simulink model "GridConnectedPV"  (R2023b)
settings: Solver=ode23t  StartTime=0.0  StopTime=simulation.timeSim  MaxStep=1/(5*solarPlant.switchFrequency)  RelTol=1e-3  AbsTol=1e-3
PreLoadFcn:
  | run('GridConnectedPVData');
undefined symbols (not defined in the file or in its folder): closedLoop, controller, grid, protection, sensor, solarPanel, solarPlant
libraries: nesl_utility x29, simulink x19, fl_lib x18, ee_lib x12, eeTransforms x2, simulink_extras x2, eeRmsMeasurement x1, eeSinusoidalMeasurement x1, slpidlib x1, eePwmGeneratorThreeLevel x1, eePwmGenerator x1
(part 1 of 2)
CloseFcn:
  | try,close(figHandleGridconnectedSolarThreePhase),end
  | clear figHandleGridconnectedSolarThreePhase
  | clear warnState
  | clear simlog_GridConnectedPV
  | 
  | clear solarPanel grid solarPlant sensor controller protection simulation
  | clear inductorDesign closedLoop
  | clear remainingPowerPerString
  | clear simulation  MPPT  powerCircuit
  | clear incrementalConductance perturbationAndObservation
  | clear discrete average continuous
  | clear modelName X U idx t x y X U A B C D G closedLoop
  | clear npts f G magline_h phsline_h presentMPPTVariant presentInverterVariant
  | clear i inverter twoLevel threeLevel geometricMean
  | clear currentLoopPole figAxes
  | clear xout yout tout
  | clear figHandleGridconnectedSolarthreePhase
Description:
  | Three-Phase Grid-Connected Solar Photovoltaic System
  | 
  | %
settings Model: Creator=The MathWorks, Inc.  LastModifiedBy=dy350
settings SolverCC: AlgebraicLoopSolver=TrustRegion
settings DataIOCC: SaveState=on  SignalLogging=off  DSMLogging=off  ReturnWorkspaceOutputs=off
settings OptimizationCC: ReuseModelBlockBuffer=off
settings DebuggingCC: UnconnectedInputMsg=warning  UnconnectedOutputMsg=warning  UnconnectedLineMsg=warning
settings ModelReferenceCC: EnableRefExpFcnMdlSchedulingChecks=on
settings RTWCC: DLArmComputeVersion=19.05
settings SimscapeCC: SimscapeLogType=all  SimscapeLogName=simlog_GridConnectedPV  SimscapeLogLimitData=off

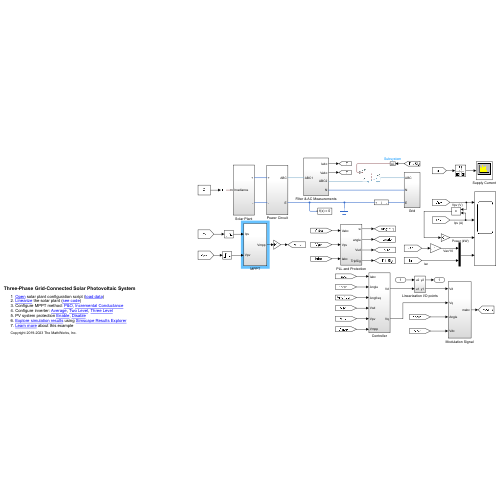
[thumbnail: Simulink's stored preview of the top-level diagram]
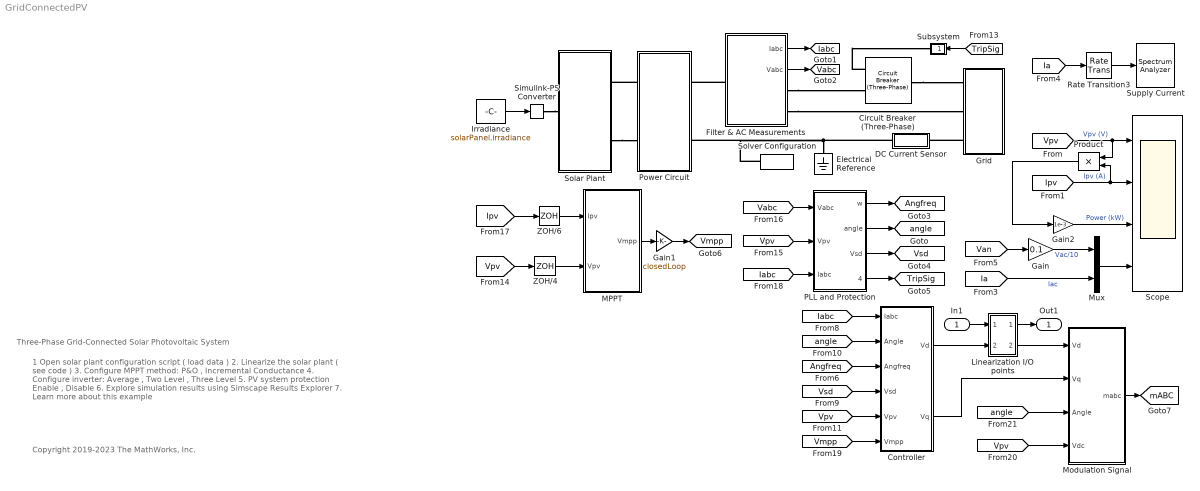
== system GridConnectedPV ==
  note: 1 Open solar plant configuration script ( load data )
      | 2. Linearize the solar plant ( see code )
      | 3. Configure MPPT method: P&O , Incremental Conductance
      | 4. Configure inverter: Average , Two Level , Three Level
      | 5. PV system protection Enable , Disable
      | 6. Explore simulation results using Simscape Results Explorer
      | 7. Learn more about this example
  note: Three-Phase Grid-Connected Solar Photovoltaic System
  note: Copyright 2019-2023 The MathWorks, Inc.
  In1 : Inport
  Circuit Breaker (Three-Phase) : ee_lib/Switches & Breakers/Circuit Breaker (Three-Phase)  R_closed=0.0001 Ohm  G_open=1e-6 1/Ohm  threshold=0.5 V  breaker_behavior=ee.enum.switches.breakerBehavior.zeroCrossingEnable
      settings: InternalSimscapePortConfiguration="{\"Bottom\":[],\"Left\":[{\"id\":\"vT\",\"label\":\"vT\",\"type\":\"input\"},{\"id\":\"N1\",\"label\":\"~1\",\"type\":\"foundation.electrical.three_phase\"}],\"Right\":[{\"id\":\"N2\",\"label\":\"~2\",\"type\":\"foundation.electrical.three_phase\"}],\"Top\":[]}"
  Controller : Subsystem
  DC Current Sensor : Subsystem
      mask Display: disp('i')
  Electrical Reference : fl_lib/Electrical/Electrical Elements/Electrical Reference
  Filter & AC Measurements : Subsystem
  Gain : Gain  Gain=0.1
  Gain1 : Gain  Gain=closedLoop
  Gain2 : Gain  Gain=1e-3
  Grid : Subsystem
  Irradiance : Constant  Value=solarPanel.irradiance
  Linearization I/O points : Subsystem
  MPPT : Subsystem
  Modulation Signal : Subsystem
  Mux : Mux  Inputs=2
  PLL and Protection : Subsystem
  Power Circuit : Subsystem
  Product : Product
  Rate Transition3 : RateTransition  OutPortSampleTime=1/(5*solarPlant.switchFrequency)
  Scope : Scope  NumInputPorts=4
  Simulink-PS Converter : nesl_utility/Simulink-PS Converter  PhysicalDomain=network_engine_domain  SubClassName=ps_input  LeftPortType=input  RightPortType=output  PseudoPeriodic=off  Frequencies=[]  NoiseDistribution=none  NoiseParameters=[]  Unit=1  AffineConversion=off  FilteringAndDerivatives=provide  SimscapeFilterOrder=1  InputFilterTimeConstant=0.001  UdotUserProvided=0
  Solar Plant : Subsystem
  Solver Configuration : nesl_utility/Solver Configuration  PhysicalDomain=network_engine_domain  SubClassName=solver  LeftPortType=input  RightPortType=generic  Tones=[]  Harmonics=[]  SimulateNoise=off  Profile=off  UseLocalSampling=off  EnableSwitchedLinearOptims=on  FrequencyDomain=off  UseCCode=off  RelTol=0.001  AbsTol=1e-06  MinStep=1e-09  ToWorkspace=off  RevertToSquareIcSolve=off  NumHomotopyIterations=100  PhasorMode=off  PhasorModeNumHarmonics=1  ConsistencySolver=NEWTON_FTOL  IndexReductionMethod=DerivativeReplacement  DoDC=off  ResidualTolerance=1e-9  ConsistencyTolSource=GLOBAL  ConsistencyAbsTol=0.001  ConsistencyRelTol=0.001  ConsistencyTolFactor=0.001  UseLocalSolver=off  LocalSolverChoice=NE_TRAPEZOIDAL_ADVANCER  ResolveIndetEquations=on  FunctionEvalNumThread=1  LocalSolverSampleTime=1e-7  DoFixedCost=off  MaxNonlinIter=10  MaxModeIter=2  ComputeImpulses=off  ImpulseIterations=2  LinearAlgebra=auto  LinearAlgebraNumThread=0  EquationFormulation=NE_TIME_EF  DelaysMemoryBudget=1024  AutomaticFiltering=on  FilteringTimeConstant=0.001  PartitionStorageMethod=AS_NEEDED  PartitionMemoryBudget=1024  PartitionMethod=FAST  MultibodyUseLocalSolver=off  MultibodyLocalSolverChoice=ODE1  MultibodyLocalSolverSampleTime=0.001
  Subsystem : Subsystem
  Supply Current : SpectrumAnalyzer  WindowPosition=[1.000000,49.000000,1707.000000,996.000000,]  ScopeFrameLocation=window  SpectrumType=RMS  Method=Welch  SampleRate=100000  PlotAsTwoSidedSpectrum=off  FrequencyScale=Log  AxesScaling=Manual  Span=50000  CenterFrequency=25000  StartFrequency=0  StopFrequency=50000  RBWSource=Property  RBW=9  OverlapPercent=90  AveragingMethod=Running  SpectrumUnits=Vrms  YLimits=[-5.01533311,45.13799799]  ColorLimits=[0.0061790664803535039207,16.888204283875005274]  ShowLegend=on
      settings: OpenAtSimulationStart=off
  ZOH/4 : ZeroOrderHold  SampleTime=solarPlant.timeMPPT
  ZOH/6 : ZeroOrderHold  SampleTime=solarPlant.timeMPPT
  Out1 : Outport  VectorParamsAs1DForOutWhenUnconnected=off
  tag scope: Angfreq=global, Iabc=global, TripSig=global, Vabc=global, Vmpp=global, Vsd=global, angle=global, mABC=global
  wires:
  [Iabc] -> Controller/1(Iabc)
  [Vpv] -> Controller/5(Vpv)
  [Vpv] -> PLL and Protection/2(Vpv)
  In1/1 -> Linearization I/O points/1(u2)
  [Vpv] -> ZOH/4/1
  [angle] -> Modulation Signal/3(Angle)
  Linearization I/O points/1(y2) -> Out1/1
  [TripSig] -> Subsystem/1(i)
  Controller/1(Vd) -> Linearization I/O points/2(u1)
  Controller/2(Vq) -> Modulation Signal/2(Vq)
  Gain/1 -> Mux/1  "Vac/10"
  [Ipv] -> Product/2, Scope/2  "Ipv (A)"
  Filter & AC Measurements/1(Iabc) -> [Iabc]
  MPPT/1(Vmpp) -> Gain1/1
  Modulation Signal/1(mabc) -> [mABC]
  PLL and Protection/3(Vsd) -> [Vsd]
  [Vmpp] -> Controller/6(Vmpp)
  PLL and Protection/2(angle) -> [angle]
  PLL and Protection/4(TripSig) -> [TripSig]
  [Vsd] -> Controller/4(Vsd)
  Rate Transition3/1 -> Supply Current/1
  Filter & AC Measurements/2(Vabc) -> [Vabc]
  PLL and Protection/1(w) -> [Angfreq]
  [Iabc] -> PLL and Protection/3(Iabc)
  [Ia] -> Rate Transition3/1
  [Ipv] -> ZOH/6/1
  [Vpv] -> Modulation Signal/4(Vdc)
  [angle] -> Controller/2(Angle)
  [Angfreq] -> Controller/3(Angfreq)
  [Vabc] -> PLL and Protection/1(Vabc)
  [Van] -> Gain/1
  Mux/1 -> Scope/4
  Linearization I/O points/2(y1) -> Modulation Signal/1(Vd)
  Gain2/1 -> Scope/3  "Power (kW)"
  ZOH/6/1 -> MPPT/1(Ipv)
  [Ia] -> Mux/2  "Iac"
  [Vpv] -> Product/1, Scope/1  "Vpv (V)"
  Product/1 -> Gain2/1
  ZOH/4/1 -> MPPT/2(Vpv)
  Gain1/1 -> [Vmpp]
  Irradiance/1 -> Simulink-PS Converter/1
  connections:
  Electrical Reference/LConn1 -- DC Current Sensor/RConn1 -- Solver Configuration/RConn1 -- Power Circuit/RConn2
  Filter & AC Measurements/RConn1 -- Circuit Breaker (Three-Phase)/LConn2
  Filter & AC Measurements/RConn2 -- Grid/LConn2
  Filter & AC Measurements/LConn1 -- Power Circuit/RConn1
  Power Circuit/LConn1 -- Solar Plant/RConn1
  Grid/LConn3 -- DC Current Sensor/LConn1
  Solar Plant/RConn2 -- Power Circuit/LConn2
  Simulink-PS Converter/RConn1 -- Solar Plant/LConn1
  Circuit Breaker (Three-Phase)/RConn1 -- Grid/LConn1
  Circuit Breaker (Three-Phase)/LConn1 -- Subsystem/RConn1

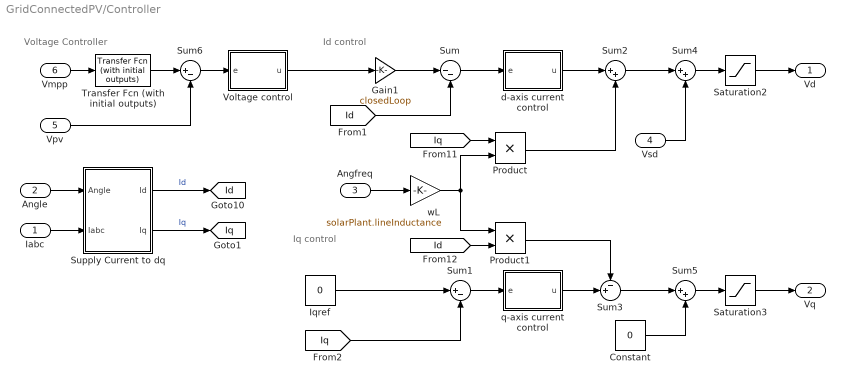
== system GridConnectedPV/Controller ==
  note: Id control
  note: Voltage Controller
  note: Iq control
  Iabc : Inport
  Angle : Inport  Port=2
  Angfreq : Inport  Port=3
  Vsd : Inport  Port=4
  Vpv : Inport  Port=5
  Vmpp : Inport  Port=6
  Constant : Constant  Value=0
  Gain1 : Gain  Gain=closedLoop
  Iqref : Constant  Value=0
  Product : Product
  Product1 : Product
  Saturation2 : Saturate  UpperLimit=controller.currentVoltMax*1.5  LowerLimit=-1*controller.currentVoltMax*1.5
  Saturation3 : Saturate  UpperLimit=controller.currentVoltMax*1.5  LowerLimit=-1*controller.currentVoltMax*1.5
  Sum : Sum  Inputs=|--
  Sum1 : Sum  Inputs=|+-
  Sum2 : Sum  Inputs=|++
  Sum3 : Sum  Inputs=-+|
  Sum4 : Sum  Inputs=|++
  Sum5 : Sum  Inputs=|++
  Sum6 : Sum  Inputs=|+-
  Supply Current to dq : Subsystem
  Transfer Fcn (with initial outputs) : simulink_extras/Additional Linear/Transfer Fcn (with initial outputs)  N=[1]  D="[solarPlant.timeMPPT*50  1]"  Y0=solarPlant.DCMPPTValue  U0=solarPlant.DCMPPTValue
  Voltage control : Subsystem
  d-axis current control : Subsystem
  q-axis current control : Subsystem
  wL : Gain  Gain=solarPlant.lineInductance
  Vd : Outport  VectorParamsAs1DForOutWhenUnconnected=off
  Vq : Outport  Port=2  VectorParamsAs1DForOutWhenUnconnected=off
  tag scope: Id=global, Iq=global
  wires:
  Sum1/1 -> q-axis current control/1(e)
  wL/1 -> Product/2, Product1/1
  [Id] -> Product1/2
  [Iq] -> Product/1
  Product1/1 -> Sum3/1
  Product/1 -> Sum2/2
  Sum3/1 -> Sum5/1
  Sum2/1 -> Sum4/1
  Sum4/1 -> Saturation2/1
  Sum5/1 -> Saturation3/1
  Angfreq/1 -> wL/1
  Constant/1 -> Sum5/2
  Angle/1 -> Supply Current to dq/1(Angle)
  Vpv/1 -> Sum6/2
  Sum/1 -> d-axis current control/1(e)
  [Id] -> Sum/2
  d-axis current control/1(u) -> Sum2/1
  q-axis current control/1(u) -> Sum3/2
  Supply Current to dq/1(Id) -> [Id]  "Id"
  Supply Current to dq/2(Iq) -> [Iq]  "Iq"
  Iabc/1 -> Supply Current to dq/2(Iabc)
  Vsd/1 -> Sum4/2
  Sum6/1 -> Voltage control/1(e)
  Vmpp/1 -> Transfer Fcn (with initial outputs)/1
  Transfer Fcn (with initial outputs)/1 -> Sum6/1
  Saturation3/1 -> Vq/1
  Saturation2/1 -> Vd/1
  Iqref/1 -> Sum1/1
  [Iq] -> Sum1/2
  Voltage control/1(u) -> Gain1/1
  Gain1/1 -> Sum/1

== system GridConnectedPV/DC Current Sensor ==
  note: In the transformerless grid connected PV system, leakage current depends on, PWM technique, DC bus voltage ripple, earth resistance and semi conductor switch switching time. So for accurately estimating the leakage current requires better PWM technique (bipolar PWM), DC bus voltage ripple, semi conductor model and earth resistance.
  Current Sensor : fl_lib/Electrical/Electrical Sensors/Current Sensor
      settings: LogSimulationData=on
  PS-Simulink Converter : nesl_utility/PS-Simulink Converter  PhysicalDomain=network_engine_domain  SubClassName=ps_output  LeftPortType=input  RightPortType=output  PseudoPeriodic=off  Frequencies=[]  VectorFormat=1-D array  Unit=1  AffineConversion=off
  Scope : Scope
  Sensor dynamics : TransferFcn  Numerator=1  Denominator=[1/sensor.samplingFreq 1]
  - : PMIOPort  Side=Left
  + : PMIOPort  Port=2  Side=Right
  wires:
  PS-Simulink Converter/1 -> Sensor dynamics/1
  Sensor dynamics/1 -> Scope/1
  connections:
  Current Sensor/RConn2 -- -/RConn1
  +/RConn1 -- Current Sensor/LConn1
  Current Sensor/RConn1 -- PS-Simulink Converter/LConn1

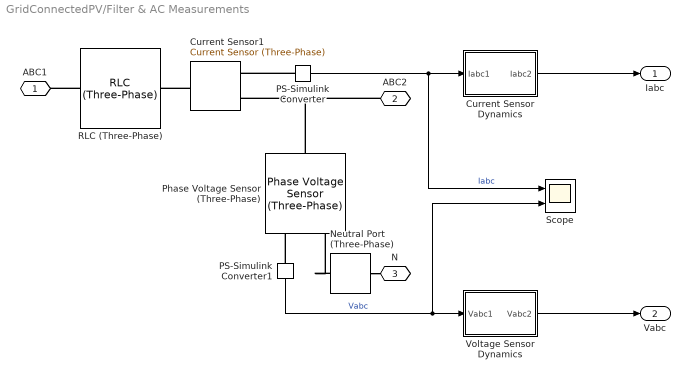
== system GridConnectedPV/Filter & AC Measurements ==
  Current Sensor Dynamics : Subsystem
  Current Sensor1 : ee_lib/Sensors & Transducers/Current Sensor (Three-Phase)
  Neutral Port (Three-Phase) : ee_lib/Connectors & References/Neutral Port (Three-Phase)  G_parasitic=1e-12 1/Ohm
      settings: InternalSimscapePortConfiguration="{\"Bottom\":[],\"Left\":[{\"id\":\"N\",\"label\":\"~\",\"type\":\"foundation.electrical.three_phase\"}],\"Right\":[{\"id\":\"n\",\"label\":\"n\",\"type\":\"foundation.electrical.electrical\"}],\"Top\":[]}"
  PS-Simulink Converter : nesl_utility/PS-Simulink Converter  PhysicalDomain=network_engine_domain  SubClassName=ps_output  LeftPortType=input  RightPortType=output  PseudoPeriodic=off  Frequencies=[]  VectorFormat=1-D array  Unit=inherit  AffineConversion=off
  PS-Simulink Converter1 : nesl_utility/PS-Simulink Converter  PhysicalDomain=network_engine_domain  SubClassName=ps_output  LeftPortType=input  RightPortType=output  PseudoPeriodic=off  Frequencies=[]  VectorFormat=1-D array  Unit=inherit  AffineConversion=off
  Phase Voltage Sensor (Three-Phase) : ee_lib/Sensors & Transducers/Phase Voltage Sensor (Three-Phase)
  RLC (Three-Phase) : ee_lib/Passive/RLC Assemblies/RLC (Three-Phase)  component_structure=4  R=solarPlant.inductorResistance Ohm  L=solarPlant.lineInductance H  C=1e-6 F  R_parasitic=1e-6 Ohm  G_parasitic=1e-6 1/Ohm  IL_specify=on  IL_priority=High  IL=[0, 0, 0] A  IL_nominal_specify=off  IL_nominal_unit=A  IL_nominal_value=1  VC_specify=on  VC_priority=High  VC=[0, 0, 0] V  VC_nominal_specify=off  VC_nominal_unit=V  VC_nominal_value=1
      settings: InternalSimscapePortConfiguration="{\"Bottom\":[],\"Left\":[{\"id\":\"N1\",\"label\":\"~1\",\"type\":\"foundation.electrical.three_phase\"}],\"Right\":[{\"id\":\"N2\",\"label\":\"~2\",\"type\":\"foundation.electrical.three_phase\"}],\"Top\":[]}"
  Scope : Scope  NumInputPorts=2
  Voltage Sensor Dynamics : Subsystem
  ABC1 : PMIOPort  Side=Left
  ABC2 : PMIOPort  Port=2  Side=Right
  N : PMIOPort  Port=3  Side=Right
  Iabc : Outport
  Vabc : Outport  Port=2
  wires:
  PS-Simulink Converter/1 -> Scope/1, Current Sensor Dynamics/1(Iabc1)  "Iabc"
  Current Sensor Dynamics/1(Iabc2) -> Iabc/1
  Voltage Sensor Dynamics/1(Vabc2) -> Vabc/1
  PS-Simulink Converter1/1 -> Scope/2, Voltage Sensor Dynamics/1(Vabc1)  "Vabc"
  connections:
  Current Sensor1/LConn1 -- RLC (Three-Phase)/RConn1
  Phase Voltage Sensor (Three-Phase)/LConn1 -- ABC2/RConn1 -- Current Sensor1/RConn2
  PS-Simulink Converter/LConn1 -- Current Sensor1/RConn1
  PS-Simulink Converter1/LConn1 -- Phase Voltage Sensor (Three-Phase)/RConn1
  Neutral Port (Three-Phase)/LConn1 -- Phase Voltage Sensor (Three-Phase)/RConn2
  Neutral Port (Three-Phase)/RConn1 -- N/RConn1
  RLC (Three-Phase)/LConn1 -- ABC1/RConn1

== system GridConnectedPV/Grid ==
  Resistor : fl_lib/Electrical/Electrical Elements/Resistor  R=50 Ohm  i_specify=off  i_priority=None  i=0 A  i_nominal_specify=off  i_nominal_unit=A  i_nominal_value=1  v_specify=off  v_priority=None  v=0 V  v_nominal_specify=off  v_nominal_unit=V  v_nominal_value=1
  Voltage Source (Three-Phase) : ee_lib/Sources/Voltage Source (Three-Phase)  vline_rms=grid.actualLineVoltage V  shift=0 deg  freq=grid.frequency Hz  impedance_option=0  SShortCircuit=1e6 V*A  XR=15  R=0.01 Ohm  L=3.97e-4 H  harmonic_option=0  harmonic_orders=[5, 7, 11, 13]  harmonic_ratios=[.1, .1, .1, .1]  G_parasitic=0 1/Ohm  I_specify=off  I_priority=None  I=[ 0 0 0 ] A  I_nominal_specify=off  I_nominal_unit=A  I_nominal_value=1
  ABC : PMIOPort  Side=Left
  N : PMIOPort  Port=2  Side=Left
  E : PMIOPort  Port=3  Side=Left
  connections:
  E/RConn1 -- Resistor/RConn1
  ABC/RConn1 -- Voltage Source (Three-Phase)/RConn1
  Voltage Source (Three-Phase)/LConn1 -- N/RConn1 -- Resistor/LConn1

== system GridConnectedPV/Linearization I//O points ==
  u2 : Inport
  u1 : Inport  Port=2
  "Set to 1 for closed-loop operation, and set to 0 when linearizing" : Gain  Gain=closedLoop  SaturateOnIntegerOverflow=on  OutDataTypeStr=Inherit: Same as input  ParamDataTypeStr=Inherit: Same as input
  Sum1 : Sum  Inputs=++|  InputSameDT=on  SaturateOnIntegerOverflow=on  OutDataTypeStr=Inherit: Same as first input
  y2 : Outport  VectorParamsAs1DForOutWhenUnconnected=off
  y1 : Outport  Port=2  VectorParamsAs1DForOutWhenUnconnected=off
  wires:
  Sum1/1 -> y1/1
  u2/1 -> Sum1/1
  "Set to 1 for closed-loop operation, and set to 0 when linearizing"/1 -> Sum1/2
  u1/1 -> y2/1, "Set to 1 for closed-loop operation, and set to 0 when linearizing"/1

== system GridConnectedPV/MPPT ==
  Ipv : Inport
  Vpv : Inport  Port=2
  Constant : Constant  Value=solarPlant.endMPPTValue
  MPPT Algorithm : Subsystem  Variant=on
  Switch : Switch  Threshold=solarPlant.endMPPTValue  SaturateOnIntegerOverflow=off  InputSameDT=off
  Vmpp : Outport  VectorParamsAs1DForOutWhenUnconnected=off
  tag scope: Ipvnow=global, Vpvnow=global
  wires:
  Vpv/1 -> [Vpvnow], MPPT Algorithm/2(Vpv)
  Ipv/1 -> [Ipvnow], MPPT Algorithm/1(Ipv)
  Constant/1 -> Switch/1
  MPPT Algorithm/1(Vmpp) -> Switch/3, Switch/2
  Switch/1 -> Vmpp/1

== system GridConnectedPV/Modulation Signal ==
  Vd : Inport
  Vq : Inport  Port=2
  Angle : Inport  Port=3
  Vdc : Inport  Port=4
  Gating Signal : Subsystem
  "dq to alpha beta " : Subsystem
  mabc : Outport  VectorParamsAs1DForOutWhenUnconnected=off
  wires:
  Gating Signal/1(mabc) -> mabc/1
  Vdc/1 -> Gating Signal/2(Vdc)
  "dq to alpha beta "/1(Vabc) -> Gating Signal/1(Vmod)
  Vd/1 -> "dq to alpha beta "/1("d ")
  Angle/1 -> "dq to alpha beta "/3(angle)
  Vq/1 -> "dq to alpha beta "/2(q)

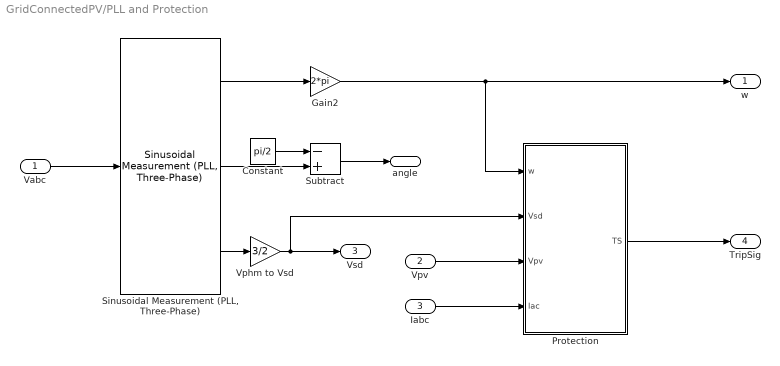
== system GridConnectedPV/PLL and Protection ==
  Vabc : Inport
  Vpv : Inport  Port=2
  Iabc : Inport  Port=3
  Constant : Constant  Value=pi/2
  Gain2 : Gain  Gain=2*pi
  Protection : Subsystem
  "Sinusoidal Measurement (PLL, Three-Phase)" : eeSinusoidalMeasurement/Sinusoidal Measurement (PLL, Three-Phase)  Kp_LF=0.05  Ki_LF=1  F0=grid.frequency  Theta0=0  Ts=0
  Subtract : Sum  Inputs=-+
  Vphm to Vsd : Gain  Gain=3/2
  w : Outport  VectorParamsAs1DForOutWhenUnconnected=off
  angle : Outport  Port=2  VectorParamsAs1DForOutWhenUnconnected=off
  Vsd : Outport  Port=3  VectorParamsAs1DForOutWhenUnconnected=off
  TripSig : Outport  Port=4  VectorParamsAs1DForOutWhenUnconnected=off
  wires:
  "Sinusoidal Measurement (PLL, Three-Phase)"/3 -> Vphm to Vsd/1
  Gain2/1 -> Protection/1(w), w/1
  "Sinusoidal Measurement (PLL, Three-Phase)"/1 -> Gain2/1
  Vabc/1 -> "Sinusoidal Measurement (PLL, Three-Phase)"/1
  Protection/1(TS) -> TripSig/1
  Vpv/1 -> Protection/3(Vpv)
  Iabc/1 -> Protection/4(Iac)
  Subtract/1 -> angle/1
  "Sinusoidal Measurement (PLL, Three-Phase)"/2 -> Subtract/2
  Constant/1 -> Subtract/1
  Vphm to Vsd/1 -> Vsd/1, Protection/2(Vsd)

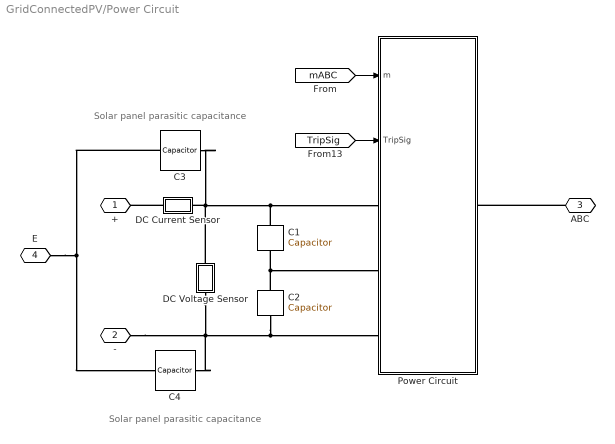
== system GridConnectedPV/Power Circuit ==
  note: Solar panel parasitic capacitance
  note: Solar panel parasitic capacitance
  C1 : fl_lib/Electrical/Electrical Elements/Capacitor  c=solarPlant.capacitance*2 F  r=1e-6 Ohm  g=0 1/Ohm  i_specify=off  i_priority=High  i=0 A  i_nominal_specify=off  i_nominal_unit=A  i_nominal_value=1  v_specify=off  v_priority=High  v=0 V  v_nominal_specify=off  v_nominal_unit=V  v_nominal_value=1  vc_specify=on  vc_priority=High  vc=solarPlant.DCMPPTValue/2 V  vc_nominal_specify=off  vc_nominal_unit=V  vc_nominal_value=1
  C2 : fl_lib/Electrical/Electrical Elements/Capacitor  c=solarPlant.capacitance*2 F  r=1e-6 Ohm  g=0 1/Ohm  i_specify=off  i_priority=High  i=0 A  i_nominal_specify=off  i_nominal_unit=A  i_nominal_value=1  v_specify=off  v_priority=High  v=0 V  v_nominal_specify=off  v_nominal_unit=V  v_nominal_value=1  vc_specify=on  vc_priority=High  vc=solarPlant.DCMPPTValue/2 V  vc_nominal_specify=off  vc_nominal_unit=V  vc_nominal_value=1
  C3 : fl_lib/Electrical/Electrical Elements/Capacitor  c=solarPlant.parasiticCapacitance/2 F  r=1 Ohm  g=0 1/Ohm  i_specify=off  i_priority=High  i=0 A  i_nominal_specify=off  i_nominal_unit=A  i_nominal_value=1  v_specify=off  v_priority=High  v=0 V  v_nominal_specify=off  v_nominal_unit=V  v_nominal_value=1  vc_specify=on  vc_priority=High  vc=solarPlant.DCMPPTValue V  vc_nominal_specify=off  vc_nominal_unit=V  vc_nominal_value=1
  C4 : fl_lib/Electrical/Electrical Elements/Capacitor  c=solarPlant.parasiticCapacitance/2 F  r=1 Ohm  g=0 1/Ohm  i_specify=off  i_priority=High  i=0 A  i_nominal_specify=off  i_nominal_unit=A  i_nominal_value=1  v_specify=off  v_priority=High  v=0 V  v_nominal_specify=off  v_nominal_unit=V  v_nominal_value=1  vc_specify=on  vc_priority=High  vc=solarPlant.DCMPPTValue V  vc_nominal_specify=off  vc_nominal_unit=V  vc_nominal_value=1
  DC Current Sensor : Subsystem
      mask Display: disp('i')
  DC Voltage Sensor : Subsystem
      mask Display: disp('v');
  Power Circuit : Subsystem  Variant=on  VariantControl=Variant1
  + : PMIOPort  Side=Left
  - : PMIOPort  Port=2  Side=Left
  ABC : PMIOPort  Port=3  Side=Right
  E : PMIOPort  Port=4  Side=Right
  wires:
  [mABC] -> Power Circuit/1(m)
  [TripSig] -> Power Circuit/2(TripSig)
  connections:
  -/RConn1 -- DC Voltage Sensor/LConn1 -- C4/LConn1 -- Power Circuit/LConn3 -- C2/RConn1
  C2/LConn1 -- Power Circuit/LConn2 -- C1/RConn1
  DC Current Sensor/LConn1 -- C3/LConn1 -- Power Circuit/LConn1 -- C1/LConn1 -- DC Voltage Sensor/RConn1
  DC Current Sensor/RConn1 -- +/RConn1
  C3/RConn1 -- E/RConn1 -- C4/RConn1
  ABC/RConn1 -- Power Circuit/RConn1

== system GridConnectedPV/Solar Plant ==
  Current-Controlled Current Source- Scale panel current to Np parallel strings : fl_lib/Electrical/Electrical Sources/Current-Controlled Current Source  K=-1*(solarPlant.numParallelPanel-1)  i1_specify=off  i1_priority=None  i1=0 A  i1_nominal_specify=off  i1_nominal_unit=A  i1_nominal_value=1  i2_specify=off  i2_priority=None  i2=0 A  i2_nominal_specify=off  i2_nominal_unit=A  i2_nominal_value=1
      settings: InternalSimscapePortConfiguration="{\"Bottom\":[],\"Left\":[{\"id\":\"p1\",\"label\":\"+\",\"type\":\"foundation.electrical.electrical\"},{\"id\":\"head\",\"label\":\"\",\"type\":\"foundation.electrical.electrical\"}],\"Right\":[{\"id\":\"n1\",\"label\":\"-\",\"type\":\"foundation.electrical.electrical\"},{\"id\":\"tail\",\"label\":\"\",\"type\":\"foundation.electrical.electrical\"}],\"Top\":[]}"
  Solar Panel : Subsystem  mask(Solar Panel){}
      mask help: Models a solar panel using a parallel-connected sting of solar cells. The solar cell strings are modeled using a single Solar Cell block from the Simscape(TM) Electrical(TM) Sources library.
      mask Display: image('SolarPanelValidationIcon.jpg')
  Voltage-Controlled Voltage Source - Scale panel voltage to Ns series panel : fl_lib/Electrical/Electrical Sources/Voltage-Controlled Voltage Source  K=-1*(solarPlant.numSeriesPanel-1)  v1_specify=off  v1_priority=None  v1=0 V  v1_nominal_specify=off  v1_nominal_unit=V  v1_nominal_value=1  v2_specify=off  v2_priority=None  v2=0 V  v2_nominal_specify=off  v2_nominal_unit=V  v2_nominal_value=1
      settings: InternalSimscapePortConfiguration="{\"Bottom\":[],\"Left\":[{\"id\":\"p1\",\"label\":\"+\",\"type\":\"foundation.electrical.electrical\"},{\"id\":\"p2\",\"label\":\"+\",\"type\":\"foundation.electrical.electrical\"}],\"Right\":[{\"id\":\"n1\",\"label\":\"-\",\"type\":\"foundation.electrical.electrical\"},{\"id\":\"n2\",\"label\":\"-\",\"type\":\"foundation.electrical.electrical\"}],\"Top\":[]}"
  + : PMIOPort  Side=Right
  Irradiance : PMIOPort  Port=2  Side=Left
  - : PMIOPort  Port=3  Side=Right
  connections:
  Voltage-Controlled Voltage Source - Scale panel voltage to Ns series panel/RConn2 -- Voltage-Controlled Voltage Source - Scale panel voltage to Ns series panel/RConn1 -- Solar Panel/RConn1
  Voltage-Controlled Voltage Source - Scale panel voltage to Ns series panel/LConn1 -- Current-Controlled Current Source- Scale panel current to Np parallel strings/LConn2 -- -/RConn1 -- Solar Panel/RConn2
  Current-Controlled Current Source- Scale panel current to Np parallel strings/RConn1 -- Current-Controlled Current Source- Scale panel current to Np parallel strings/RConn2 -- +/RConn1
  Current-Controlled Current Source- Scale panel current to Np parallel strings/LConn1 -- Voltage-Controlled Voltage Source - Scale panel voltage to Ns series panel/LConn2
  Solar Panel/LConn1 -- Irradiance/RConn1

== system GridConnectedPV/Subsystem ==
  i : Inport
  Data Type Conversion : DataTypeConversion  SaturateOnIntegerOverflow=off  RndMeth=Floor
  Simulink-PS Converter : nesl_utility/Simulink-PS Converter  PhysicalDomain=network_engine_domain  SubClassName=ps_input  LeftPortType=input  RightPortType=output  PseudoPeriodic=off  Frequencies=[]  NoiseDistribution=none  NoiseParameters=[]  Unit=1  AffineConversion=off  FilteringAndDerivatives=provide  SimscapeFilterOrder=1  InputFilterTimeConstant=0.001  UdotUserProvided=0
  o : PMIOPort  Side=Right
  wires:
  Data Type Conversion/1 -> Simulink-PS Converter/1
  i/1 -> Data Type Conversion/1
  connections:
  Simulink-PS Converter/RConn1 -- o/RConn1

== system GridConnectedPV/Controller/Supply Current to dq ==
  Angle : Inport
  Iabc : Inport  Port=2
  Demux : Demux  Outputs=3
  Filter : TransferFcn  Denominator=[1e-5 1]
  Filter1 : TransferFcn  Denominator=[1e-5 1]
  Park Transform : eeTransforms/Park Transform  AxisAlignment=D-axis  PowerInvariant=off
  Terminator : Terminator
  Id : Outport  VectorParamsAs1DForOutWhenUnconnected=off
  Iq : Outport  Port=2  VectorParamsAs1DForOutWhenUnconnected=off
  wires:
  Demux/1 -> Filter/1
  Park Transform/1 -> Demux/1
  Demux/3 -> Terminator/1
  Filter/1 -> Id/1
  Filter1/1 -> Iq/1
  Demux/2 -> Filter1/1
  Iabc/1 -> Park Transform/1
  Angle/1 -> Park Transform/2

== system GridConnectedPV/Controller/Voltage control ==
  e : Inport
  Integrator : Integrator  LimitOutput=on  UpperSaturationLimit=solarPlant.maxPowerACCurrent*sqrt(2)*3/2*1.3  LowerSaturationLimit=-solarPlant.maxPowerACCurrent*sqrt(2)*3/2*1.3
  Ki : Gain  Gain=1/controller.voltagePole
  Kp : Gain  Gain=controller.voltageGain
  Saturation : Saturate  UpperLimit=solarPlant.maxPowerACCurrent*sqrt(2)*3/2*1.3  LowerLimit=-1*solarPlant.maxPowerACCurrent*sqrt(2)*3/2*1.3
  Sum7 : Sum  Inputs=|++
  u : Outport  VectorParamsAs1DForOutWhenUnconnected=off
  wires:
  Integrator/1 -> Sum7/2
  Saturation/1 -> u/1
  Sum7/1 -> Saturation/1
  e/1 -> Kp/1
  Kp/1 -> Ki/1, Sum7/1
  Ki/1 -> Integrator/1

== system GridConnectedPV/Controller/d-axis current control ==
  e : Inport
  Integrator : Integrator  LimitOutput=on  UpperSaturationLimit=controller.currentVoltMax  LowerSaturationLimit=-controller.currentVoltMax
  Ki : Gain  Gain=1/controller.currentPole
  Kp : Gain  Gain=controller.currentGain
  Saturation : Saturate  UpperLimit=controller.currentVoltMax  LowerLimit=-1*controller.currentVoltMax
  Sum7 : Sum  Inputs=|++
  u : Outport  VectorParamsAs1DForOutWhenUnconnected=off
  wires:
  Integrator/1 -> Sum7/2
  Saturation/1 -> u/1
  Sum7/1 -> Saturation/1
  e/1 -> Kp/1
  Kp/1 -> Ki/1, Sum7/1
  Ki/1 -> Integrator/1

== system GridConnectedPV/Controller/q-axis current control ==
  e : Inport
  Integrator : Integrator  LimitOutput=on  UpperSaturationLimit=controller.currentVoltMax  LowerSaturationLimit=-controller.currentVoltMax
  Ki : Gain  Gain=1/controller.currentPole
  Kp : Gain  Gain=controller.currentGain
  Saturation : Saturate  UpperLimit=controller.currentVoltMax  LowerLimit=-1*controller.currentVoltMax
  Sum7 : Sum  Inputs=|++
  u : Outport  VectorParamsAs1DForOutWhenUnconnected=off
  wires:
  Ki/1 -> Integrator/1
  Kp/1 -> Sum7/1, Ki/1
  e/1 -> Kp/1
  Sum7/1 -> Saturation/1
  Saturation/1 -> u/1
  Integrator/1 -> Sum7/2

== system GridConnectedPV/Filter & AC Measurements/Current Sensor Dynamics ==
  Iabc1 : Inport
  Demux : Demux  Outputs=3
  Mux : Mux  Inputs=3
  Sensor dynamics2 : TransferFcn  Numerator=1  Denominator=[1/sensor.samplingFreq 1]
  Sensor dynamics3 : TransferFcn  Numerator=1  Denominator=[1/sensor.samplingFreq 1]
  Sensor dynamics4 : TransferFcn  Numerator=1  Denominator=[1/sensor.samplingFreq 1]
  Iabc2 : Outport
  tag scope: Ia=global
  wires:
  Iabc1/1 -> Demux/1
  Sensor dynamics3/1 -> Mux/2
  Mux/1 -> Iabc2/1
  Sensor dynamics2/1 -> [Ia], Mux/1
  Demux/1 -> Sensor dynamics2/1
  Demux/3 -> Sensor dynamics4/1
  Demux/2 -> Sensor dynamics3/1
  Sensor dynamics4/1 -> Mux/3

== system GridConnectedPV/Filter & AC Measurements/Voltage Sensor Dynamics ==
  Vabc1 : Inport
  Demux : Demux  Outputs=3
  Mux : Mux  Inputs=3
  Sensor dynamics2 : TransferFcn  Numerator=1  Denominator=[1/sensor.samplingFreq 1]
  Sensor dynamics3 : TransferFcn  Numerator=1  Denominator=[1/sensor.samplingFreq 1]
  Sensor dynamics4 : TransferFcn  Numerator=1  Denominator=[1/sensor.samplingFreq 1]
  Vabc2 : Outport
  tag scope: Van=global
  wires:
  Vabc1/1 -> Demux/1
  Sensor dynamics3/1 -> Mux/2
  Mux/1 -> Vabc2/1
  Sensor dynamics2/1 -> [Van], Mux/1
  Demux/1 -> Sensor dynamics2/1
  Demux/3 -> Sensor dynamics4/1
  Demux/2 -> Sensor dynamics3/1
  Sensor dynamics4/1 -> Mux/3

== system GridConnectedPV/MPPT/MPPT Algorithm ==
  Ipv : Inport
  Vpv : Inport  Port=2
  IncrementalConductance : Subsystem  VariantControl=incrementalConductance
  PerturbationAndObsrvation : Subsystem  VariantControl=perturbationAndObservation
  Vmpp : Outport  VectorParamsAs1DForOutWhenUnconnected=off

== system GridConnectedPV/Modulation Signal/Gating Signal ==
  Vmod : Inport
  Vdc : Inport  Port=2
  Normalize by DC voltage and disable if DC volts too low : Subsystem
  "[-1,1]" : Saturate  UpperLimit=1  LowerLimit=-1
  mabc : Outport  VectorParamsAs1DForOutWhenUnconnected=off
  wires:
  Normalize by DC voltage and disable if DC volts too low/1(y) -> "[-1,1]"/1
  Vdc/1 -> Normalize by DC voltage and disable if DC volts too low/2(v_dc)
  Vmod/1 -> Normalize by DC voltage and disable if DC volts too low/1(u)
  "[-1,1]"/1 -> mabc/1

== system GridConnectedPV/Modulation Signal/dq to alpha beta  ==
  "d " : Inport
  q : Inport  Port=2
  angle : Inport  Port=3
  Constant : Constant  Value=0
  Inverse Park Transform : eeTransforms/Inverse Park Transform  AxisAlignment=D-axis  PowerInvariant=off
  Mux : Mux  Inputs=3
  Vabc : Outport  VectorParamsAs1DForOutWhenUnconnected=off
  wires:
  Inverse Park Transform/1 -> Vabc/1
  angle/1 -> Inverse Park Transform/2
  Mux/1 -> Inverse Park Transform/1
  Constant/1 -> Mux/3
  q/1 -> Mux/2
  "d "/1 -> Mux/1

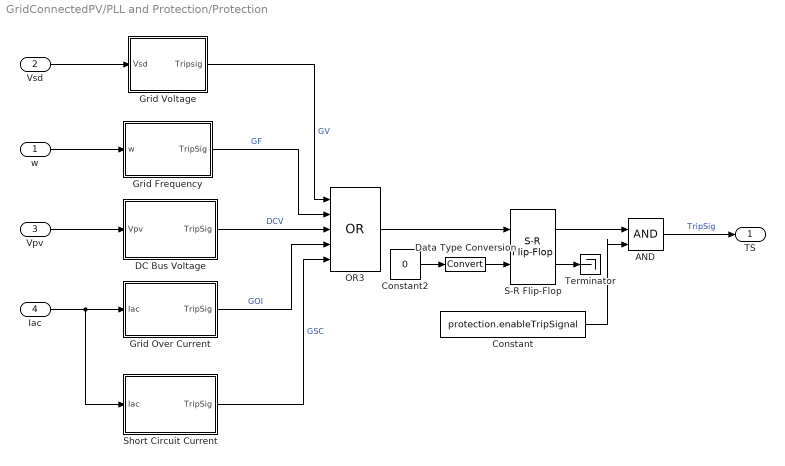
== system GridConnectedPV/PLL and Protection/Protection ==
  w : Inport
  Vsd : Inport  Port=2
  Vpv : Inport  Port=3
  Iac : Inport  Port=4
  AND : Logic  IconShape=distinctive  AllPortsSameDT=off  OutDataTypeStr=boolean
  Constant : Constant  Value=protection.enableTripSignal
  Constant2 : Constant  Value=0
  DC Bus Voltage : Subsystem
  Data Type Conversion : DataTypeConversion  SaturateOnIntegerOverflow=off  RndMeth=Floor
  Grid Frequency : Subsystem
  Grid Over Current : Subsystem
  Grid Voltage : Subsystem
  OR3 : Logic  Operator=OR  Inputs=5  IconShape=distinctive  AllPortsSameDT=off  OutDataTypeStr=boolean
  S-R Flip-Flop : simulink_extras/Flip Flops/S-R Flip-Flop  initial_condition=0
  Short Circuit Current : Subsystem
  Terminator : Terminator
  TS : Outport  VectorParamsAs1DForOutWhenUnconnected=off
  wires:
  Iac/1 -> Grid Over Current/1(Iac), Short Circuit Current/1(Iac)
  Vsd/1 -> Grid Voltage/1(Vsd)
  Grid Voltage/1(Tripsig) -> OR3/1  "GV"
  w/1 -> Grid Frequency/1(w)
  Grid Frequency/1(TripSig) -> OR3/2  "GF"
  Vpv/1 -> DC Bus Voltage/1(Vpv)
  DC Bus Voltage/1(TripSig) -> OR3/3  "DCV"
  Grid Over Current/1(TripSig) -> OR3/4  "GOI"
  Short Circuit Current/1(TripSig) -> OR3/5  "GSC"
  Constant/1 -> AND/2
  AND/1 -> TS/1  "TripSig"
  OR3/1 -> S-R Flip-Flop/1
  S-R Flip-Flop/1 -> AND/1
  Data Type Conversion/1 -> S-R Flip-Flop/2
  Constant2/1 -> Data Type Conversion/1
  S-R Flip-Flop/2 -> Terminator/1

== system GridConnectedPV/Power Circuit/DC Current Sensor ==
  Current Sensor : fl_lib/Electrical/Electrical Sensors/Current Sensor
      settings: LogSimulationData=on
  PS-Simulink Converter : nesl_utility/PS-Simulink Converter  PhysicalDomain=network_engine_domain  SubClassName=ps_output  LeftPortType=input  RightPortType=output  PseudoPeriodic=off  Frequencies=[]  VectorFormat=1-D array  Unit=1  AffineConversion=off
  Sensor dynamics : TransferFcn  Numerator=1  Denominator=[1/sensor.samplingFreq 1]
  - : PMIOPort  Side=Left
  + : PMIOPort  Port=2  Side=Right
  tag scope: Ipv=global
  wires:
  PS-Simulink Converter/1 -> Sensor dynamics/1
  Sensor dynamics/1 -> [Ipv]
  connections:
  Current Sensor/RConn2 -- -/RConn1
  +/RConn1 -- Current Sensor/LConn1
  Current Sensor/RConn1 -- PS-Simulink Converter/LConn1

== system GridConnectedPV/Power Circuit/DC Voltage Sensor ==
  PS-Simulink Converter : nesl_utility/PS-Simulink Converter  PhysicalDomain=network_engine_domain  SubClassName=ps_output  LeftPortType=input  RightPortType=output  PseudoPeriodic=off  Frequencies=[]  VectorFormat=1-D array  Unit=1  AffineConversion=off
  Sensor dynamics : TransferFcn  Numerator=1  Denominator=[1/sensor.samplingFreq 1]
  Voltage Sensor : fl_lib/Electrical/Electrical Sensors/Voltage Sensor
      settings: LogSimulationData=on
  - : PMIOPort  Side=Left
  + : PMIOPort  Port=2  Side=Right
  tag scope: Vpv=global
  wires:
  PS-Simulink Converter/1 -> Sensor dynamics/1
  Sensor dynamics/1 -> [Vpv]
  connections:
  Voltage Sensor/LConn1 -- +/RConn1
  Voltage Sensor/RConn1 -- PS-Simulink Converter/LConn1
  Voltage Sensor/RConn2 -- -/RConn1

== system GridConnectedPV/Power Circuit/Power Circuit ==
  m : Inport
  TripSig : Inport  Port=2
  Average : Subsystem  VariantControl=average
  Three Level : Subsystem  VariantControl=threeLevel
  Two Level : Subsystem  VariantControl=twoLevel
  + : PMIOPort  Side=Left
  O : PMIOPort  Port=2  Side=Left
  - : PMIOPort  Port=3  Side=Left
  ABC : PMIOPort  Port=4  Side=Right

== system GridConnectedPV/Solar Plant/Solar Panel ==
  Current-Controlled Current Source : fl_lib/Electrical/Electrical Sources/Current-Controlled Current Source  K=-1*(solarPanel.numParallelCell-1)  i1_specify=off  i1_priority=None  i1=0 A  i1_nominal_specify=off  i1_nominal_unit=A  i1_nominal_value=1  i2_specify=off  i2_priority=None  i2=0 A  i2_nominal_specify=off  i2_nominal_unit=A  i2_nominal_value=1
      settings: InternalSimscapePortConfiguration="{\"Bottom\":[],\"Left\":[{\"id\":\"p1\",\"label\":\"+\",\"type\":\"foundation.electrical.electrical\"},{\"id\":\"head\",\"label\":\"\",\"type\":\"foundation.electrical.electrical\"}],\"Right\":[{\"id\":\"n1\",\"label\":\"-\",\"type\":\"foundation.electrical.electrical\"},{\"id\":\"tail\",\"label\":\"\",\"type\":\"foundation.electrical.electrical\"}],\"Top\":[]}"
  Solar Cell : ee_lib/Sources/Solar Cell  prm=1  Isc=solarPanel.shortCircuitCurrentPV/solarPanel.numParallelCell A  Voc=solarPanel.openCircuitVoltagePV/solarPanel.numSeriesCell V  Is=1e-6 A  Is2=0 A  Iph=7.34 A  Ir0=solarPanel.irradianceMeasurement W/m^2  ec=solarPanel.qualityFactor  N2=2  Rs=solarPanel.seriesResistance Ohm  Rp=inf Ohm  N_series=solarPanel.numSeriesCell-1  N_parallel=1  TIPH1=solarPanel.currentTemperatureCoeff 1/K  EG=1.11 eV  TXIS1=solarPanel.temperatureExponent  TXIS2=3  TRS1=0  TRP1=0  Tmeas=solarPanel.temperatureMeasurement degC  TFIXED=solarPanel.temperature degC  thermal_mass=100 J/K  initial_temperature=25 degC
  Ir : PMIOPort  Side=Left
  + : PMIOPort  Port=2  Side=Right
  - : PMIOPort  Port=3  Side=Right
  connections:
  Current-Controlled Current Source/LConn2 -- -/RConn1 -- Solar Cell/RConn1
  Ir/RConn1 -- Solar Cell/LConn1
  Current-Controlled Current Source/LConn1 -- Solar Cell/LConn2
  Current-Controlled Current Source/RConn1 -- Current-Controlled Current Source/RConn2 -- +/RConn1

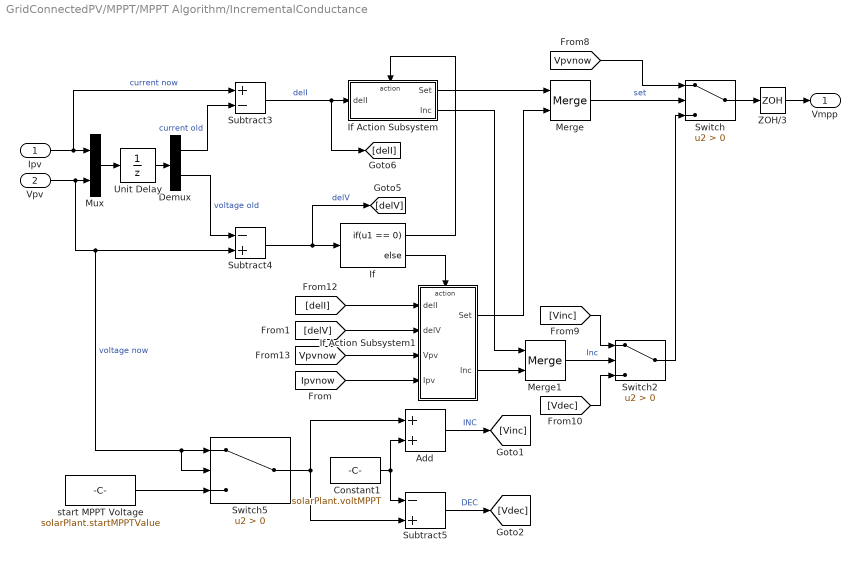
== system GridConnectedPV/MPPT/MPPT Algorithm/IncrementalConductance ==
  Ipv : Inport
  Vpv : Inport  Port=2
  Add : Sum
  Constant1 : Constant  Value=solarPlant.voltMPPT
  Demux : Demux  Outputs=2
  If : If  IfExpression=u1 == 0
  If Action Subsystem : Subsystem  TreatAsAtomicUnit=on
  If Action Subsystem1 : Subsystem  TreatAsAtomicUnit=on
  Merge : Merge
  Merge1 : Merge
  Mux : Mux  Inputs=2
  Subtract3 : Sum  Inputs=+-
  Subtract4 : Sum  Inputs=-+
  Subtract5 : Sum  Inputs=-+
  Switch : Switch  Criteria=u2 > Threshold  SaturateOnIntegerOverflow=off  InputSameDT=off
  Switch2 : Switch  Criteria=u2 > Threshold  SaturateOnIntegerOverflow=off  InputSameDT=off
  Switch5 : Switch  Criteria=u2 > Threshold  SaturateOnIntegerOverflow=off  InputSameDT=off
  Unit Delay : UnitDelay  InitialCondition=solarPlant.startMPPTValue  SampleTime=solarPlant.timeMPPT  HasFrameUpgradeWarning=on
  ZOH/3 : ZeroOrderHold  SampleTime=solarPlant.timeMPPT
  start MPPT Voltage : Constant  Value=solarPlant.startMPPTValue
  Vmpp : Outport  VectorParamsAs1DForOutWhenUnconnected=off
  wires:
  Merge1/1 -> Switch2/2  "Inc"
  [Vpvnow] -> Switch/1
  If Action Subsystem1/2(Inc) -> Merge1/2
  If Action Subsystem/2(Inc) -> Merge1/1
  If/2 -> If Action Subsystem1/Action
  If Action Subsystem/1(Set) -> Merge/1
  [delV] -> If Action Subsystem1/2(delV)
  [delI] -> If Action Subsystem1/1(delI)
  Merge/1 -> Switch/2  "set"
  If Action Subsystem1/1(Set) -> Merge/2
  If/1 -> If Action Subsystem/Action
  [Vpvnow] -> If Action Subsystem1/3(Vpv)
  Switch2/1 -> Switch/3
  [Ipvnow] -> If Action Subsystem1/4(Ipv)
  Ipv/1 -> Mux/1, Subtract3/1  "current now"
  Unit Delay/1 -> Demux/1
  Mux/1 -> Unit Delay/1
  Vpv/1 -> Subtract4/2, Switch5/2, Switch5/1, Mux/2  "voltage now"
  Demux/2 -> Subtract4/1  "voltage old"
  Demux/1 -> Subtract3/2  "current old"
  Subtract3/1 -> [delI], If Action Subsystem/1(delI)  "delI"
  Subtract4/1 -> [delV], If/1  "delV"
  [Vinc] -> Switch2/1
  [Vdec] -> Switch2/3
  Switch/1 -> ZOH/3/1
  ZOH/3/1 -> Vmpp/1
  Switch5/1 -> Add/1, Subtract5/2
  Subtract5/1 -> [Vdec]  "DEC"
  start MPPT Voltage/1 -> Switch5/3
  Constant1/1 -> Add/2, Subtract5/1
  Add/1 -> [Vinc]  "INC"

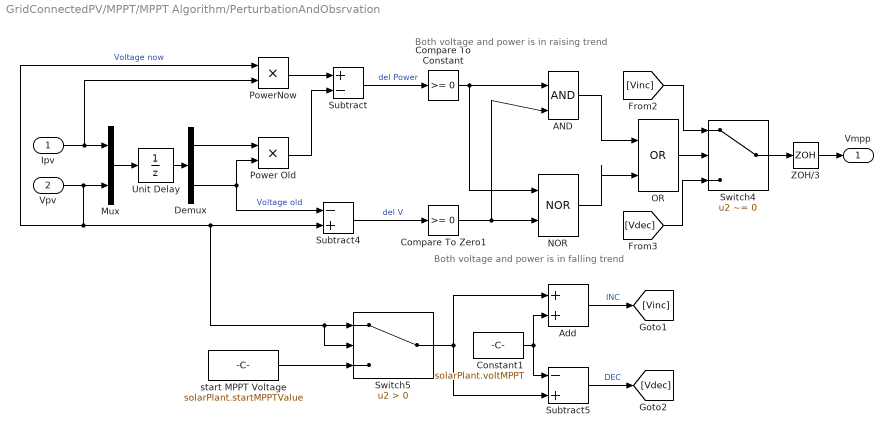
== system GridConnectedPV/MPPT/MPPT Algorithm/PerturbationAndObsrvation ==
  note: Both voltage and power is in raising trend
  note: Both voltage and power is in falling trend
  Ipv : Inport
  Vpv : Inport  Port=2
  AND : Logic  IconShape=distinctive  AllPortsSameDT=off  OutDataTypeStr=boolean
  Add : Sum
  Compare To Constant : simulink/Logic and Bit Operations/Compare To Constant  relop=>=  const=0  OutDataTypeStr=boolean
  Compare To Zero1 : simulink/Logic and Bit Operations/Compare To Zero  relop=>=  OutDataTypeStr=boolean
  Constant1 : Constant  Value=solarPlant.voltMPPT
  Demux : Demux  Outputs=2
  Mux : Mux  Inputs=2
  NOR : Logic  Operator=NOR  IconShape=distinctive  AllPortsSameDT=off  OutDataTypeStr=boolean
  OR : Logic  Operator=OR  IconShape=distinctive  AllPortsSameDT=off  OutDataTypeStr=boolean
  Power Old : Product
  PowerNow : Product
  Subtract : Sum  Inputs=+-
  Subtract4 : Sum  Inputs=-+
  Subtract5 : Sum  Inputs=-+
  Switch4 : Switch  Criteria=u2 ~= 0  SaturateOnIntegerOverflow=off  InputSameDT=off
  Switch5 : Switch  Criteria=u2 > Threshold  SaturateOnIntegerOverflow=off  InputSameDT=off
  Unit Delay : UnitDelay  InitialCondition=solarPlant.startMPPTValue  SampleTime=solarPlant.timeMPPT  HasFrameUpgradeWarning=on
  ZOH/3 : ZeroOrderHold  SampleTime=solarPlant.timeMPPT
  start MPPT Voltage : Constant  Value=solarPlant.startMPPTValue
  Vmpp : Outport  VectorParamsAs1DForOutWhenUnconnected=off
  wires:
  NOR/1 -> OR/2
  OR/1 -> Switch4/2
  Compare To Zero1/1 -> NOR/2, AND/2
  AND/1 -> OR/1
  Compare To Constant/1 -> AND/1, NOR/1
  Mux/1 -> Unit Delay/1
  Ipv/1 -> PowerNow/2, Mux/1
  Demux/1 -> Power Old/1
  Unit Delay/1 -> Demux/1
  Demux/2 -> Power Old/2, Subtract4/1  "Voltage old"
  Vpv/1 -> Switch5/2, Switch5/1, Subtract4/2, PowerNow/1, Mux/2  "Voltage now"
  PowerNow/1 -> Subtract/1
  Power Old/1 -> Subtract/2
  Subtract4/1 -> Compare To Zero1/1  "del V"
  Subtract/1 -> Compare To Constant/1  "del Power"
  [Vdec] -> Switch4/3
  [Vinc] -> Switch4/1
  Switch4/1 -> ZOH/3/1
  ZOH/3/1 -> Vmpp/1
  Switch5/1 -> Add/1, Subtract5/2
  Subtract5/1 -> [Vdec]  "DEC"
  start MPPT Voltage/1 -> Switch5/3
  Constant1/1 -> Add/2, Subtract5/1
  Add/1 -> [Vinc]  "INC"

== system GridConnectedPV/Modulation Signal/Gating Signal/Normalize by DC voltage and disable if DC volts too low ==
  u : Inport
  v_dc : Inport  Port=2
  Min DC voltage : Constant  Value=0.5*solarPlant.startMPPTValue
  Product1 : Product  Inputs=*/  InputSameDT=on  SaturateOnIntegerOverflow=on  OutDataTypeStr=Inherit: Same as first input
  Switch1 : Switch  Threshold=0.5*solarPlant.maxPowerVoltage  SaturateOnIntegerOverflow=off
  y : Outport  VectorParamsAs1DForOutWhenUnconnected=off
  wires:
  Min DC voltage/1 -> Switch1/3
  Switch1/1 -> Product1/2
  v_dc/1 -> Switch1/2, Switch1/1
  u/1 -> Product1/1
  Product1/1 -> y/1

== system GridConnectedPV/PLL and Protection/Protection/DC Bus Voltage ==
  Vpv : Inport
  Compare To Constant5 : simulink/Logic and Bit Operations/Compare To Constant  relop=>  const=protection.dcBusVoltageTripTime  OutDataTypeStr=boolean
  Compare To Constant6 : simulink/Logic and Bit Operations/Compare To Constant  relop=>  const=protection.dcBusMaxVoltage  OutDataTypeStr=boolean
  Compare To Constant7 : simulink/Logic and Bit Operations/Compare To Constant  relop=<  const=protection.dcBusMinVoltage  OutDataTypeStr=boolean
  Data Type Conversion1 : DataTypeConversion  SaturateOnIntegerOverflow=off  RndMeth=Floor
  Integrator1 : Integrator  ExternalReset=falling
  OR2 : Logic  Operator=OR  IconShape=distinctive  AllPortsSameDT=off  OutDataTypeStr=boolean
  Transfer Fcn2 : TransferFcn  Denominator=[1e-4 1]
  TripSig : Outport  VectorParamsAs1DForOutWhenUnconnected=off
  wires:
  Compare To Constant6/1 -> OR2/2
  Transfer Fcn2/1 -> Compare To Constant6/1, Compare To Constant7/1
  Compare To Constant7/1 -> OR2/1
  Vpv/1 -> Transfer Fcn2/1
  Integrator1/1 -> Compare To Constant5/1
  Data Type Conversion1/1 -> Integrator1/2, Integrator1/1
  OR2/1 -> Data Type Conversion1/1
  Compare To Constant5/1 -> TripSig/1

== system GridConnectedPV/PLL and Protection/Protection/Grid Frequency ==
  w : Inport
  Compare To Constant2 : simulink/Logic and Bit Operations/Compare To Constant  relop=>  const=protection.gridMaxFreq*2*pi  OutDataTypeStr=boolean
  Compare To Constant3 : simulink/Logic and Bit Operations/Compare To Constant  relop=<  const=protection.gridMinFreq*2*pi  OutDataTypeStr=boolean
  Compare To Constant5 : simulink/Logic and Bit Operations/Compare To Constant  relop=>  const=protection.gridFrequencyTripTime  OutDataTypeStr=boolean
  Data Type Conversion1 : DataTypeConversion  SaturateOnIntegerOverflow=off  RndMeth=Floor
  Integrator1 : Integrator  ExternalReset=falling
  OR1 : Logic  Operator=OR  IconShape=distinctive  AllPortsSameDT=off  OutDataTypeStr=boolean
  Transfer Fcn1 : TransferFcn  Denominator=[1e-2 1]
  TripSig : Outport  VectorParamsAs1DForOutWhenUnconnected=off
  wires:
  Compare To Constant5/1 -> TripSig/1
  Transfer Fcn1/1 -> Compare To Constant2/1, Compare To Constant3/1
  Data Type Conversion1/1 -> Integrator1/2, Integrator1/1
  w/1 -> Transfer Fcn1/1
  Integrator1/1 -> Compare To Constant5/1
  OR1/1 -> Data Type Conversion1/1
  Compare To Constant2/1 -> OR1/1
  Compare To Constant3/1 -> OR1/2

== system GridConnectedPV/PLL and Protection/Protection/Grid Over Current ==
  Iac : Inport
  Compare To Constant8 : simulink/Logic and Bit Operations/Compare To Constant  relop=>  const=protection.overLoadCurrentTripTime  OutDataTypeStr=boolean
  Compare To Constant9 : simulink/Logic and Bit Operations/Compare To Constant  relop=>  const=protection.overLoadCurrent  OutDataTypeStr=boolean
  Data Type Conversion3 : DataTypeConversion  SaturateOnIntegerOverflow=off  RndMeth=Floor
  Demux : Demux  Outputs=3
  Integrator2 : Integrator  ExternalReset=falling
  OR : Logic  Operator=OR  Inputs=3  IconShape=distinctive  AllPortsSameDT=off  OutDataTypeStr=boolean
  RMS Measurement : eeRmsMeasurement/RMS Measurement  LabelModeActiveChoice=Total  F=grid.frequency  SpecifyHarmonics=off  K=[0 1 2]  Ts=1/(20*grid.frequency)
  TripSig : Outport  VectorParamsAs1DForOutWhenUnconnected=off
  wires:
  Compare To Constant9/1 -> Data Type Conversion3/1
  Data Type Conversion3/1 -> Integrator2/2, Integrator2/1
  Integrator2/1 -> Compare To Constant8/1
  Iac/1 -> RMS Measurement/1
  RMS Measurement/1 -> Compare To Constant9/1
  Demux/1 -> OR/1
  Demux/2 -> OR/2
  Demux/3 -> OR/3
  OR/1 -> TripSig/1
  Compare To Constant8/1 -> Demux/1

== system GridConnectedPV/PLL and Protection/Protection/Grid Voltage ==
  Vsd : Inport
  Compare To Constant : simulink/Logic and Bit Operations/Compare To Constant  relop=>  const=protection.gridMaxVoltage*3/2  OutDataTypeStr=boolean
  Compare To Constant1 : simulink/Logic and Bit Operations/Compare To Constant  relop=<  const=protection.gridMinVoltage*3/2  OutDataTypeStr=boolean
  Compare To Constant4 : simulink/Logic and Bit Operations/Compare To Constant  relop=>  const=protection.gridVoltageTripTime  OutDataTypeStr=boolean
  Data Type Conversion : DataTypeConversion  SaturateOnIntegerOverflow=off  RndMeth=Floor
  Integrator : Integrator  ExternalReset=falling
  OR : Logic  Operator=OR  IconShape=distinctive  AllPortsSameDT=off  OutDataTypeStr=boolean
  Transfer Fcn : TransferFcn  Denominator=[1e-3 1]
  Tripsig : Outport  VectorParamsAs1DForOutWhenUnconnected=off
  wires:
  OR/1 -> Data Type Conversion/1
  Data Type Conversion/1 -> Integrator/2, Integrator/1
  Transfer Fcn/1 -> Compare To Constant/1, Compare To Constant1/1
  Vsd/1 -> Transfer Fcn/1
  Integrator/1 -> Compare To Constant4/1
  Compare To Constant1/1 -> OR/1
  Compare To Constant/1 -> OR/2
  Compare To Constant4/1 -> Tripsig/1

== system GridConnectedPV/PLL and Protection/Protection/Short Circuit Current ==
  Iac : Inport
  AND : Logic  IconShape=distinctive  AllPortsSameDT=off  OutDataTypeStr=boolean
  Abs : Abs  SaturateOnIntegerOverflow=off
  Clock : Clock
  Compare To Constant : simulink/Logic and Bit Operations/Compare To Constant  relop=>  const=protection.shortCircuitCurrentStartTime  OutDataTypeStr=boolean
  Compare To Constant11 : simulink/Logic and Bit Operations/Compare To Constant  relop=>  const=protection.shortCircuitCurrent  OutDataTypeStr=boolean
  Demux : Demux  Outputs=3
  OR : Logic  Operator=OR  Inputs=3  IconShape=distinctive  AllPortsSameDT=off  OutDataTypeStr=boolean
  TripSig : Outport  VectorParamsAs1DForOutWhenUnconnected=off
  wires:
  Compare To Constant11/1 -> AND/1
  Iac/1 -> Abs/1
  Abs/1 -> Compare To Constant11/1
  Clock/1 -> Compare To Constant/1
  Compare To Constant/1 -> AND/2
  Demux/2 -> OR/2
  Demux/3 -> OR/3
  Demux/1 -> OR/1
  OR/1 -> TripSig/1
  AND/1 -> Demux/1

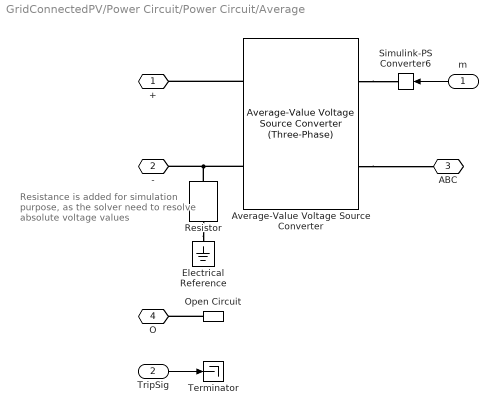
== system GridConnectedPV/Power Circuit/Power Circuit/Average ==
  note: Resistance is added for simulation purpose, as the solver need to resolve absolute voltage values
  m : Inport
  TripSig : Inport  Port=2
  Average-Value Voltage Source Converter : ee_lib/Semiconductors & Converters/Converters/Average-Value Voltage Source Converter (Three-Phase)  port_option=ee.enum.threePhasePort.composite  frequency_option=ee.enum.converters.frequency.variable  FRated=60 Hz  losses_parameterization=ee.enum.converters.losses.fixed  Pfixed=1 W  ks=0.01  kc1=1.7 V  kc2=0.01 Ohm  Ploss_vect=[100, 800, 1870, 3250, 4900] W  Irms_vect=[10, 100, 200, 300, 400] A  Vdc_nom=300 V  thermal_mass=30000 J/K  temperature_specify=off  temperature_priority=High  temperature=298.15 K  temperature_nominal_specify=off  temperature_nominal_unit=K  temperature_nominal_value=1
      settings: InternalSimscapePortConfiguration="{\"Bottom\":[],\"Left\":[{\"id\":\"ModWave\",\"label\":\"ModWave\",\"type\":\"input\"},{\"id\":\"N\",\"label\":\"~\",\"type\":\"foundation.electrical.three_phase\"}],\"Right\":[{\"id\":\"p\",\"label\":\"+\",\"type\":\"foundation.electrical.electrical\"},{\"id\":\"n\",\"label\":\"-\",\"type\":\"foundation.electrical.electrical\"}],\"Top\":[]}"
  Electrical Reference : fl_lib/Electrical/Electrical Elements/Electrical Reference
  Open Circuit : fl_lib/Electrical/Electrical Elements/Open Circuit  v_specify=off  v_priority=None  v=0 V  v_nominal_specify=off  v_nominal_unit=V  v_nominal_value=1
  Resistor : fl_lib/Electrical/Electrical Elements/Resistor  R=1e6 Ohm  i_specify=off  i_priority=None  i=0 A  i_nominal_specify=off  i_nominal_unit=A  i_nominal_value=1  v_specify=off  v_priority=None  v=0 V  v_nominal_specify=off  v_nominal_unit=V  v_nominal_value=1
  Simulink-PS Converter6 : nesl_utility/Simulink-PS Converter  PhysicalDomain=network_engine_domain  SubClassName=ps_input  LeftPortType=input  RightPortType=output  PseudoPeriodic=off  Frequencies=[]  NoiseDistribution=none  NoiseParameters=[]  Unit=1  AffineConversion=off  FilteringAndDerivatives=provide  SimscapeFilterOrder=1  InputFilterTimeConstant=0.001  UdotUserProvided=0
  Terminator : Terminator
  + : PMIOPort  Side=Left
  - : PMIOPort  Port=2  Side=Left
  ABC : PMIOPort  Port=3  Side=Right
  O : PMIOPort  Port=4  Side=Left
  wires:
  TripSig/1 -> Terminator/1
  m/1 -> Simulink-PS Converter6/1
  connections:
  Average-Value Voltage Source Converter/LConn2 -- ABC/RConn1
  Average-Value Voltage Source Converter/LConn1 -- Simulink-PS Converter6/RConn1
  Average-Value Voltage Source Converter/RConn2 -- Resistor/LConn1 -- -/RConn1
  Average-Value Voltage Source Converter/RConn1 -- +/RConn1
  Open Circuit/LConn1 -- O/RConn1
  Resistor/RConn1 -- Electrical Reference/LConn1
